simulink model "fmcw_sim"  (R2021b)
settings: Solver=VariableStepAuto  StartTime=0.0  StopTime=0.5  RelTol=1e-3
undefined symbols (not defined in the file or in its folder): paramRadarHardwareFMCW, paramRadarWaveformFMCW
libraries: phasedenvlib x4, simulink x2, phasedtxrxlib x2, phaseddetectlib x1, phasedmisclib x1
settings Model: Creator=plato  LastModifiedBy=plato

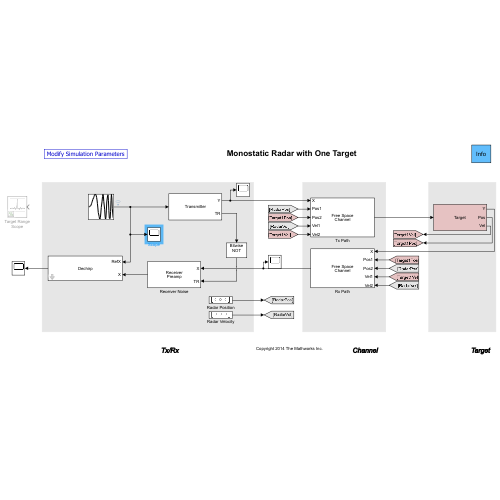
[thumbnail: Simulink's stored preview of the top-level diagram]
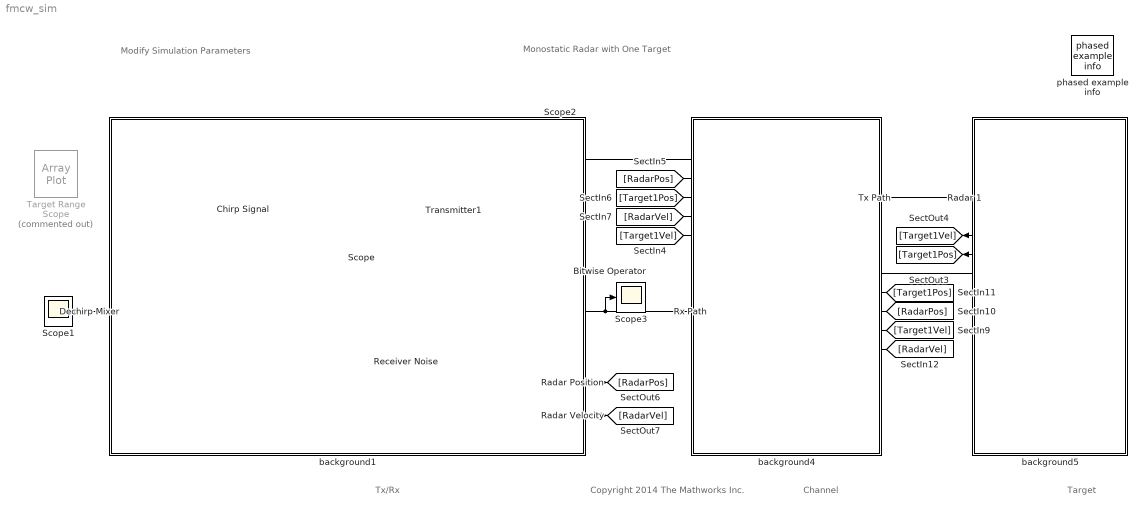
== system fmcw_sim ==
  note: Channel
  note: Copyright 2014 The Mathworks Inc.
  note: Tx/Rx
  note: Target
  note: Modify Simulation Parameters
  note: Monostatic Radar with One Target
  Bitwise Operator : simulink/Logic and Bit Operations/Bitwise Operator  logicop=NOT  UseBitMask=off  BitMask=bin2dec('11011001')  BitMaskRealWorld=Stored Integer
  Chirp Signal : simulink/Sources/Chirp Signal  f1=paramRadarWaveformFMCW.StartF  T=paramRadarWaveformFMCW.T  f2=paramRadarWaveformFMCW.EndF  VectorParams1D=off
  Dechirp Mixer : phaseddetectlib/Dechirp Mixer
      settings: SourceProductBaseCode=AR
  Radar 1 : Subsystem
      mask Display:
      | disp('Target')
      | port_label('output',1,'Y');
      | port_label('output',2,'Pos');
      | port_label('output',3,'Vel');
  Radar Position : Constant  Value=[ 0; 0; 0 ]  SampleTime=[-1, 0]
  Radar Velocity : Constant  Value=[ 0; 0; 0 ]  SampleTime=[-1, 0]
  Receiver Noise : phasedtxrxlib/Receiver Preamp  Gain=20  LossFactor=0  NoiseMethod=Noise temperature  NoiseFigure=0  ReferenceTemperature=290  SampleRateFromInputCheckbox=off  SampleRate=paramRadarWaveformFMCW.Fs  NoisePower=0  EnableInputPort=on  PhaseNoiseInputPort=off  SeedSource=Auto  Seed=0  SimulateUsing=Interpreted execution
      settings: SourceProductBaseCode=AR
  Rx Path : phasedenvlib/Free Space  PropagationSpeed=paramEnvironment.propSpeed  OperatingFrequency=paramRadarHardwareFMCW.Fc  TwoWayPropagation=off  SampleRateFromInputCheckbox=off  SampleRate=paramRadarWaveformFMCW.Fs  MaximumDistanceSource=Property  MaximumDistance=2  MaximumNumInputSamplesSource=Auto  MaximumNumInputSamples=1000  SimulateUsing=Interpreted execution
      settings: SourceProductBaseCode=AR
  Scope{,1..3} (4 alike) : Scope
  Target Range Scope : ArrayPlot  Commented=on  WindowPosition=[2478.000000,31.000000,808.000000,454.000000,]  SampleIncrement=paramRadar.metersPerSample  XOffset=paramRadar.rangeOffset  PlotType=Line  AxesScaling=Manual  MaximizeAxes=Off  Title=Radar Return  XLabel=Range (m)  YLimits=[-4.2427e-08,1.7395e-06]
  Transmitter1 : phasedtxrxlib/Transmitter  PeakPower=paramRadarHardwareFMCW.Ppow  Gain=paramRadarHardwareFMCW.TxGain  LossFactor=0  InUseOutputPort=on  CoherentOnTransmit=on  PhaseNoiseOutputPort=off  SeedSource=Auto  Seed=0  SimulateUsing=Interpreted execution
      settings: SourceProductBaseCode=AR
  Tx Path : phasedenvlib/Free Space  PropagationSpeed=paramEnvironment.propSpeed  OperatingFrequency=paramRadarHardwareFMCW.Fc  TwoWayPropagation=off  SampleRateFromInputCheckbox=off  SampleRate=paramRadarWaveformFMCW.Fs  MaximumDistanceSource=Property  MaximumDistance=2  MaximumNumInputSamplesSource=Auto  MaximumNumInputSamples=1000  SimulateUsing=Interpreted execution
      settings: SourceProductBaseCode=AR
  background1 : Subsystem  Description=Jammer
      mask Display: disp('')
  background4 : Subsystem  Description=Jammer
      mask Display: disp('')
  background5 : Subsystem  Description=Jammer
      mask Display: disp('')
  phased example info : phasedmisclib/phased example info  SystemSampleTime=-1  VariantActivationTime=update diagram  Latency=0  AutoFrameSizeCalculation=off
      settings: SourceProductBaseCode=AR
  wires:
  Transmitter1/1 -> Scope2/1, Tx Path/1
  Receiver Noise/1 -> Dechirp Mixer/2
  [RadarPos] -> Tx Path/2
  [RadarPos] -> Rx Path/3
  Radar 1/3(V) -> [Target1Vel]
  [RadarVel] -> Tx Path/4
  Radar 1/1(Out1) -> Rx Path/1
  Rx Path/1 -> Scope3/1, Receiver Noise/1
  [RadarVel] -> Rx Path/5
  [Target1Vel] -> Rx Path/4
  Transmitter1/2 -> Bitwise Operator/1
  [Target1Pos] -> Tx Path/3
  [Target1Vel] -> Tx Path/5
  Tx Path/1 -> Radar 1/1(In1)
  Chirp Signal/1 -> Dechirp Mixer/1, Scope/1, Transmitter1/1
  Radar Velocity/1 -> [RadarVel]
  Bitwise Operator/1 -> Receiver Noise/2
  Radar Position/1 -> [RadarPos]
  [Target1Pos] -> Rx Path/2
  Radar 1/2(P) -> [Target1Pos]
  Dechirp Mixer/1 -> Scope1/1

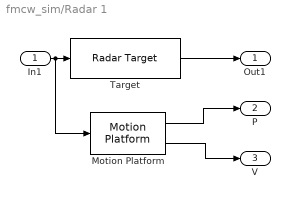
== system fmcw_sim/Radar 1 ==
  In1 : Inport
  Motion Platform : phasedenvlib/Motion Platform  MotionModel=Velocity  InitialPosition=paramGeometryFMCW.CarPos  InitialVelocity=[ 0; 0; 0 ]  VelocitySource=Property  Velocity=paramGeometryFMCW.CarVel  AccelerationSource=Property  Acceleration=[0;0;0]  CustomTrajectory=[ 0, 0, 0, 0, 0, 0, 0; 1, 0, 0, 0, 0, 0, 0 ]  ScanMode=None  InitialScanAngle=0  AzimuthSpan=[ -60, 60 ]  AzimuthScanRate=10  InitialOrientationAxes=eye( 3 )  OrientationAxesOutputPort=off  ElapsedTimeSource=Derive from reference input port  SampleRateFromInputCheckbox=off  SampleRate=paramRadarWaveformFMCW.Fs  SimulateUsing=Interpreted execution
      settings: SourceProductBaseCode=AR
  Target : phasedenvlib/Radar Target  EnablePolarization=off  Mode=Monostatic  MeanRCSSource=Property  ScatteringMatrixSource=Property  MeanRCS=paramRadarHardwareFMCW.RCS  ScatteringMatrix=eye( 2 )  Model=Nonfluctuating  PropagationSpeed=paramEnvironment.propSpeed  OperatingFrequency=paramRadarHardwareFMCW.Fc  SeedSource=Auto  Seed=0  SimulateUsing=Interpreted execution
      settings: SourceProductBaseCode=AR
  Out1 : Outport  VectorParamsAs1DForOutWhenUnconnected=off
  P : Outport  Port=2  VectorParamsAs1DForOutWhenUnconnected=off
  V : Outport  Port=3  VectorParamsAs1DForOutWhenUnconnected=off
  wires:
  Target/1 -> Out1/1
  Motion Platform/1 -> P/1
  Motion Platform/2 -> V/1
  In1/1 -> Motion Platform/1, Target/1

== system fmcw_sim/background1 ==

== system fmcw_sim/background4 ==

== system fmcw_sim/background5 ==
